simulink model "AccelerationValidation"  (R2022b)
settings: Solver=VariableStepAuto  StartTime=0.0  StopTime=10.0  RelTol=1e-3
(part 2 of 2)

== matlab function AccelerationValidation/MATLAB Function ==
  data: q input; AF output; qdot input; qdd input
function AF = forward_acceleration_kinematics(q, qdot, qdd)

q1 = q(1);
q2 = q(2);
q3 = q(3);
q4 = q(4);
q1dot = qdot(1);
q2dot = qdot(2);
q3dot = qdot(3);
q4dot = qdot(4);
q1dd = qdd(1);
q2dd = qdd(2);
q3dd = qdd(3);
q4dd = qdd(4);

J =[150*sin(q2)*sin(q1 - pi/2)*sin(q4 - pi/2) - 150*cos(q4 - pi/2)*(cos(q1 - pi/2)*sin(q3 - pi/2) + cos(q2)*cos(q3 - pi/2)*sin(q1 - pi/2)) - 185*sin(q2)*sin(q1 - pi/2),                                                                                                                                                                                                                                                                      -cos(q1 - pi/2)*(150*cos(q2)*sin(q4 - pi/2) - 185*cos(q2) + 150*cos(q3 - pi/2)*cos(q4 - pi/2)*sin(q2)),                                                                                             - cos(q2)*(185*sin(q2)*sin(q1 - pi/2) + 150*cos(q4 - pi/2)*(cos(q1 - pi/2)*sin(q3 - pi/2) + cos(q2)*cos(q3 - pi/2)*sin(q1 - pi/2)) - 150*sin(q2)*sin(q1 - pi/2)*sin(q4 - pi/2)) - sin(q2)*sin(q1 - pi/2)*(150*cos(q2)*sin(q4 - pi/2) - 185*cos(q2) + 150*cos(q3 - pi/2)*cos(q4 - pi/2)*sin(q2)),                                                                                                                - (150*cos(q2)*sin(q4 - pi/2) + 150*cos(q3 - pi/2)*cos(q4 - pi/2)*sin(q2))*(cos(q1 - pi/2)*cos(q3 - pi/2) - cos(q2)*sin(q1 - pi/2)*sin(q3 - pi/2)) - sin(q2)*sin(q3 - pi/2)*(150*cos(q4 - pi/2)*(cos(q1 - pi/2)*sin(q3 - pi/2) + cos(q2)*cos(q3 - pi/2)*sin(q1 - pi/2)) - 150*sin(q2)*sin(q1 - pi/2)*sin(q4 - pi/2));
185*cos(q1 - pi/2)*sin(q2) - 150*cos(q4 - pi/2)*(sin(q1 - pi/2)*sin(q3 - pi/2) - cos(q2)*cos(q1 - pi/2)*cos(q3 - pi/2)) - 150*cos(q1 - pi/2)*sin(q2)*sin(q4 - pi/2),                                                                                                                                                                                                                                                                      -sin(q1 - pi/2)*(150*cos(q2)*sin(q4 - pi/2) - 185*cos(q2) + 150*cos(q3 - pi/2)*cos(q4 - pi/2)*sin(q2)),                                                                                               cos(q1 - pi/2)*sin(q2)*(150*cos(q2)*sin(q4 - pi/2) - 185*cos(q2) + 150*cos(q3 - pi/2)*cos(q4 - pi/2)*sin(q2)) - cos(q2)*(150*cos(q4 - pi/2)*(sin(q1 - pi/2)*sin(q3 - pi/2) - cos(q2)*cos(q1 - pi/2)*cos(q3 - pi/2)) - 185*cos(q1 - pi/2)*sin(q2) + 150*cos(q1 - pi/2)*sin(q2)*sin(q4 - pi/2)),                                                                                                                - (150*cos(q2)*sin(q4 - pi/2) + 150*cos(q3 - pi/2)*cos(q4 - pi/2)*sin(q2))*(cos(q3 - pi/2)*sin(q1 - pi/2) + cos(q2)*cos(q1 - pi/2)*sin(q3 - pi/2)) - sin(q2)*sin(q3 - pi/2)*(150*cos(q4 - pi/2)*(sin(q1 - pi/2)*sin(q3 - pi/2) - cos(q2)*cos(q1 - pi/2)*cos(q3 - pi/2)) + 150*cos(q1 - pi/2)*sin(q2)*sin(q4 - pi/2));
                                                                                                                                                                  0, cos(q1 - pi/2)*(150*cos(q4 - pi/2)*(sin(q1 - pi/2)*sin(q3 - pi/2) - cos(q2)*cos(q1 - pi/2)*cos(q3 - pi/2)) - 185*cos(q1 - pi/2)*sin(q2) + 150*cos(q1 - pi/2)*sin(q2)*sin(q4 - pi/2)) - sin(q1 - pi/2)*(185*sin(q2)*sin(q1 - pi/2) + 150*cos(q4 - pi/2)*(cos(q1 - pi/2)*sin(q3 - pi/2) + cos(q2)*cos(q3 - pi/2)*sin(q1 - pi/2)) - 150*sin(q2)*sin(q1 - pi/2)*sin(q4 - pi/2)), sin(q2)*sin(q1 - pi/2)*(150*cos(q4 - pi/2)*(sin(q1 - pi/2)*sin(q3 - pi/2) - cos(q2)*cos(q1 - pi/2)*cos(q3 - pi/2)) - 185*cos(q1 - pi/2)*sin(q2) + 150*cos(q1 - pi/2)*sin(q2)*sin(q4 - pi/2)) + cos(q1 - pi/2)*sin(q2)*(185*sin(q2)*sin(q1 - pi/2) + 150*cos(q4 - pi/2)*(cos(q1 - pi/2)*sin(q3 - pi/2) + cos(q2)*cos(q3 - pi/2)*sin(q1 - pi/2)) - 150*sin(q2)*sin(q1 - pi/2)*sin(q4 - pi/2)), (150*cos(q4 - pi/2)*(sin(q1 - pi/2)*sin(q3 - pi/2) - cos(q2)*cos(q1 - pi/2)*cos(q3 - pi/2)) + 150*cos(q1 - pi/2)*sin(q2)*sin(q4 - pi/2))*(cos(q1 - pi/2)*cos(q3 - pi/2) - cos(q2)*sin(q1 - pi/2)*sin(q3 - pi/2)) - (150*cos(q4 - pi/2)*(cos(q1 - pi/2)*sin(q3 - pi/2) + cos(q2)*cos(q3 - pi/2)*sin(q1 - pi/2)) - 150*sin(q2)*sin(q1 - pi/2)*sin(q4 - pi/2))*(cos(q3 - pi/2)*sin(q1 - pi/2) + cos(q2)*cos(q1 - pi/2)*sin(q3 - pi/2));
                                                                                                                                                                  0,                                                                                                                                                                                                                                                                                                                                                             -sin(q1 - pi/2),                                                                                                                                                                                                                                                                                                                                                                      cos(q1 - pi/2)*sin(q2),                                                                                                                                                                                                                                                                                                                                                             - cos(q3 - pi/2)*sin(q1 - pi/2) - cos(q2)*cos(q1 - pi/2)*sin(q3 - pi/2);
                                                                                                                                                                  0,                                                                                                                                                                                                                                                                                                                                                              cos(q1 - pi/2),                                                                                                                                                                                                                                                                                                                                                                      sin(q2)*sin(q1 - pi/2),                                                                                                                                                                                                                                                                                                                                                               cos(q1 - pi/2)*cos(q3 - pi/2) - cos(q2)*sin(q1 - pi/2)*sin(q3 - pi/2);                                                                                                                                                                  1,                                                                                                                                                                                                                                                                                                                                                                           0,                                                                                                                                                                                                                                                                                                                                                                                     cos(q2),                                                                                                                                                                                                                                                                                                                                                                                                              sin(q2)*sin(q3 - pi/2)];
 
J_dot = [q4dot*(150*sin(q4 - pi/2)*(cos(q1 - pi/2)*sin(q3 - pi/2) + cos(q2)*cos(q3 - pi/2)*sin(q1 - pi/2)) + 150*cos(q4 - pi/2)*sin(q2)*sin(q1 - pi/2)) + q1dot*(150*cos(q4 - pi/2)*(sin(q1 - pi/2)*sin(q3 - pi/2) - cos(q2)*cos(q1 - pi/2)*cos(q3 - pi/2)) - 185*cos(q1 - pi/2)*sin(q2) + 150*cos(q1 - pi/2)*sin(q2)*sin(q4 - pi/2)) + q2dot*(150*cos(q2)*sin(q1 - pi/2)*sin(q4 - pi/2) - 185*cos(q2)*sin(q1 - pi/2) + 150*cos(q3 - pi/2)*cos(q4 - pi/2)*sin(q2)*sin(q1 - pi/2)) - 150*q3dot*cos(q4 - pi/2)*(cos(q1 - pi/2)*cos(q3 - pi/2) - cos(q2)*sin(q1 - pi/2)*sin(q3 - pi/2)),                                                                                                                                                                                                                                                                                                                                                                                                                                                                                  q1dot*sin(q1 - pi/2)*(150*cos(q2)*sin(q4 - pi/2) - 185*cos(q2) + 150*cos(q3 - pi/2)*cos(q4 - pi/2)*sin(q2)) - q4dot*cos(q1 - pi/2)*(150*cos(q2)*cos(q4 - pi/2) - 150*cos(q3 - pi/2)*sin(q2)*sin(q4 - pi/2)) - q2dot*cos(q1 - pi/2)*(185*sin(q2) - 150*sin(q2)*sin(q4 - pi/2) + 150*cos(q2)*cos(q3 - pi/2)*cos(q4 - pi/2)) + 150*q3dot*cos(q1 - pi/2)*cos(q4 - pi/2)*sin(q2)*sin(q3 - pi/2),        q4dot*(cos(q2)*(150*sin(q4 - pi/2)*(cos(q1 - pi/2)*sin(q3 - pi/2) + cos(q2)*cos(q3 - pi/2)*sin(q1 - pi/2)) + 150*cos(q4 - pi/2)*sin(q2)*sin(q1 - pi/2)) - sin(q2)*sin(q1 - pi/2)*(150*cos(q2)*cos(q4 - pi/2) - 150*cos(q3 - pi/2)*sin(q2)*sin(q4 - pi/2))) - q3dot*(150*cos(q2)*cos(q4 - pi/2)*(cos(q1 - pi/2)*cos(q3 - pi/2) - cos(q2)*sin(q1 - pi/2)*sin(q3 - pi/2)) - 150*cos(q4 - pi/2)*sin(q2)^2*sin(q1 - pi/2)*sin(q3 - pi/2)) + q1dot*(cos(q2)*(150*cos(q4 - pi/2)*(sin(q1 - pi/2)*sin(q3 - pi/2) - cos(q2)*cos(q1 - pi/2)*cos(q3 - pi/2)) - 185*cos(q1 - pi/2)*sin(q2) + 150*cos(q1 - pi/2)*sin(q2)*sin(q4 - pi/2)) - cos(q1 - pi/2)*sin(q2)*(150*cos(q2)*sin(q4 - pi/2) - 185*cos(q2) + 150*cos(q3 - pi/2)*cos(q4 - pi/2)*sin(q2))) + q2dot*(cos(q2)*(150*cos(q2)*sin(q1 - pi/2)*sin(q4 - pi/2) - 185*cos(q2)*sin(q1 - pi/2) + 150*cos(q3 - pi/2)*cos(q4 - pi/2)*sin(q2)*sin(q1 - pi/2)) + sin(q2)*(185*sin(q2)*sin(q1 - pi/2) + 150*cos(q4 - pi/2)*(cos(q1 - pi/2)*sin(q3 - pi/2) + cos(q2)*cos(q3 - pi/2)*sin(q1 - pi/2)) - 150*sin(q2)*sin(q1 - pi/2)*sin(q4 - pi/2)) - sin(q2)*sin(q1 - pi/2)*(185*sin(q2) - 150*sin(q2)*sin(q4 - pi/2) + 150*cos(q2)*cos(q3 - pi/2)*cos(q4 - pi/2)) - cos(q2)*sin(q1 - pi/2)*(150*cos(q2)*sin(q4 - pi/2) - 185*cos(q2) + 150*cos(q3 - pi/2)*cos(q4 - pi/2)*sin(q2))),                                                                    q1dot*((150*cos(q2)*sin(q4 - pi/2) + 150*cos(q3 - pi/2)*cos(q4 - pi/2)*sin(q2))*(cos(q3 - pi/2)*sin(q1 - pi/2) + cos(q2)*cos(q1 - pi/2)*sin(q3 - pi/2)) + sin(q2)*sin(q3 - pi/2)*(150*cos(q4 - pi/2)*(sin(q1 - pi/2)*sin(q3 - pi/2) - cos(q2)*cos(q1 - pi/2)*cos(q3 - pi/2)) + 150*cos(q1 - pi/2)*sin(q2)*sin(q4 - pi/2))) + q3dot*((150*cos(q2)*sin(q4 - pi/2) + 150*cos(q3 - pi/2)*cos(q4 - pi/2)*sin(q2))*(cos(q1 - pi/2)*sin(q3 - pi/2) + cos(q2)*cos(q3 - pi/2)*sin(q1 - pi/2)) - cos(q3 - pi/2)*sin(q2)*(150*cos(q4 - pi/2)*(cos(q1 - pi/2)*sin(q3 - pi/2) + cos(q2)*cos(q3 - pi/2)*sin(q1 - pi/2)) - 150*sin(q2)*sin(q1 - pi/2)*sin(q4 - pi/2))) - q4dot*((150*cos(q2)*cos(q4 - pi/2) - 150*cos(q3 - pi/2)*sin(q2)*sin(q4 - pi/2))*(cos(q1 - pi/2)*cos(q3 - pi/2) - cos(q2)*sin(q1 - pi/2)*sin(q3 - pi/2)) - sin(q2)*sin(q3 - pi/2)*(150*sin(q4 - pi/2)*(cos(q1 - pi/2)*sin(q3 - pi/2) + cos(q2)*cos(q3 - pi/2)*sin(q1 - pi/2)) + 150*cos(q4 - pi/2)*sin(q2)*sin(q1 - pi/2))) + q2dot*((150*sin(q2)*sin(q4 - pi/2) - 150*cos(q2)*cos(q3 - pi/2)*cos(q4 - pi/2))*(cos(q1 - pi/2)*cos(q3 - pi/2) - cos(q2)*sin(q1 - pi/2)*sin(q3 - pi/2)) - cos(q2)*sin(q3 - pi/2)*(150*cos(q4 - pi/2)*(cos(q1 - pi/2)*sin(q3 - pi/2) + cos(q2)*cos(q3 - pi/2)*sin(q1 - pi/2)) - 150*sin(q2)*sin(q1 - pi/2)*sin(q4 - pi/2)) + sin(q2)*sin(q3 - pi/2)*(150*cos(q2)*sin(q1 - pi/2)*sin(q4 - pi/2) + 150*cos(q3 - pi/2)*cos(q4 - pi/2)*sin(q2)*sin(q1 - pi/2)) - sin(q2)*sin(q1 - pi/2)*sin(q3 - pi/2)*(150*cos(q2)*sin(q4 - pi/2) + 150*cos(q3 - pi/2)*cos(q4 - pi/2)*sin(q2)));
q4dot*(150*sin(q4 - pi/2)*(sin(q1 - pi/2)*sin(q3 - pi/2) - cos(q2)*cos(q1 - pi/2)*cos(q3 - pi/2)) - 150*cos(q1 - pi/2)*cos(q4 - pi/2)*sin(q2)) - q2dot*(150*cos(q2)*cos(q1 - pi/2)*sin(q4 - pi/2) - 185*cos(q2)*cos(q1 - pi/2) + 150*cos(q1 - pi/2)*cos(q3 - pi/2)*cos(q4 - pi/2)*sin(q2)) - q1dot*(185*sin(q2)*sin(q1 - pi/2) + 150*cos(q4 - pi/2)*(cos(q1 - pi/2)*sin(q3 - pi/2) + cos(q2)*cos(q3 - pi/2)*sin(q1 - pi/2)) - 150*sin(q2)*sin(q1 - pi/2)*sin(q4 - pi/2)) - 150*q3dot*cos(q4 - pi/2)*(cos(q3 - pi/2)*sin(q1 - pi/2) + cos(q2)*cos(q1 - pi/2)*sin(q3 - pi/2)),                                                                                                                                                                                                                                                                                                                                                                                                                                                                                  150*q3dot*cos(q4 - pi/2)*sin(q2)*sin(q1 - pi/2)*sin(q3 - pi/2) - q1dot*cos(q1 - pi/2)*(150*cos(q2)*sin(q4 - pi/2) - 185*cos(q2) + 150*cos(q3 - pi/2)*cos(q4 - pi/2)*sin(q2)) - q2dot*sin(q1 - pi/2)*(185*sin(q2) - 150*sin(q2)*sin(q4 - pi/2) + 150*cos(q2)*cos(q3 - pi/2)*cos(q4 - pi/2)) - q4dot*sin(q1 - pi/2)*(150*cos(q2)*cos(q4 - pi/2) - 150*cos(q3 - pi/2)*sin(q2)*sin(q4 - pi/2)),        q2dot*(sin(q2)*(150*cos(q4 - pi/2)*(sin(q1 - pi/2)*sin(q3 - pi/2) - cos(q2)*cos(q1 - pi/2)*cos(q3 - pi/2)) - 185*cos(q1 - pi/2)*sin(q2) + 150*cos(q1 - pi/2)*sin(q2)*sin(q4 - pi/2)) - cos(q2)*(150*cos(q2)*cos(q1 - pi/2)*sin(q4 - pi/2) - 185*cos(q2)*cos(q1 - pi/2) + 150*cos(q1 - pi/2)*cos(q3 - pi/2)*cos(q4 - pi/2)*sin(q2)) + cos(q2)*cos(q1 - pi/2)*(150*cos(q2)*sin(q4 - pi/2) - 185*cos(q2) + 150*cos(q3 - pi/2)*cos(q4 - pi/2)*sin(q2)) + cos(q1 - pi/2)*sin(q2)*(185*sin(q2) - 150*sin(q2)*sin(q4 - pi/2) + 150*cos(q2)*cos(q3 - pi/2)*cos(q4 - pi/2))) - q3dot*(150*cos(q2)*cos(q4 - pi/2)*(cos(q3 - pi/2)*sin(q1 - pi/2) + cos(q2)*cos(q1 - pi/2)*sin(q3 - pi/2)) + 150*cos(q1 - pi/2)*cos(q4 - pi/2)*sin(q2)^2*sin(q3 - pi/2)) - q1dot*(cos(q2)*(185*sin(q2)*sin(q1 - pi/2) + 150*cos(q4 - pi/2)*(cos(q1 - pi/2)*sin(q3 - pi/2) + cos(q2)*cos(q3 - pi/2)*sin(q1 - pi/2)) - 150*sin(q2)*sin(q1 - pi/2)*sin(q4 - pi/2)) + sin(q2)*sin(q1 - pi/2)*(150*cos(q2)*sin(q4 - pi/2) - 185*cos(q2) + 150*cos(q3 - pi/2)*cos(q4 - pi/2)*sin(q2))) + q4dot*(cos(q2)*(150*sin(q4 - pi/2)*(sin(q1 - pi/2)*sin(q3 - pi/2) - cos(q2)*cos(q1 - pi/2)*cos(q3 - pi/2)) - 150*cos(q1 - pi/2)*cos(q4 - pi/2)*sin(q2)) + cos(q1 - pi/2)*sin(q2)*(150*cos(q2)*cos(q4 - pi/2) - 150*cos(q3 - pi/2)*sin(q2)*sin(q4 - pi/2))),                                                                    q3dot*((150*cos(q2)*sin(q4 - pi/2) + 150*cos(q3 - pi/2)*cos(q4 - pi/2)*sin(q2))*(sin(q1 - pi/2)*sin(q3 - pi/2) - cos(q2)*cos(q1 - pi/2)*cos(q3 - pi/2)) - cos(q3 - pi/2)*sin(q2)*(150*cos(q4 - pi/2)*(sin(q1 - pi/2)*sin(q3 - pi/2) - cos(q2)*cos(q1 - pi/2)*cos(q3 - pi/2)) + 150*cos(q1 - pi/2)*sin(q2)*sin(q4 - pi/2))) - q4dot*((150*cos(q2)*cos(q4 - pi/2) - 150*cos(q3 - pi/2)*sin(q2)*sin(q4 - pi/2))*(cos(q3 - pi/2)*sin(q1 - pi/2) + cos(q2)*cos(q1 - pi/2)*sin(q3 - pi/2)) - sin(q2)*sin(q3 - pi/2)*(150*sin(q4 - pi/2)*(sin(q1 - pi/2)*sin(q3 - pi/2) - cos(q2)*cos(q1 - pi/2)*cos(q3 - pi/2)) - 150*cos(q1 - pi/2)*cos(q4 - pi/2)*sin(q2))) - q1dot*((150*cos(q2)*sin(q4 - pi/2) + 150*cos(q3 - pi/2)*cos(q4 - pi/2)*sin(q2))*(cos(q1 - pi/2)*cos(q3 - pi/2) - cos(q2)*sin(q1 - pi/2)*sin(q3 - pi/2)) + sin(q2)*sin(q3 - pi/2)*(150*cos(q4 - pi/2)*(cos(q1 - pi/2)*sin(q3 - pi/2) + cos(q2)*cos(q3 - pi/2)*sin(q1 - pi/2)) - 150*sin(q2)*sin(q1 - pi/2)*sin(q4 - pi/2))) + q2dot*((150*sin(q2)*sin(q4 - pi/2) - 150*cos(q2)*cos(q3 - pi/2)*cos(q4 - pi/2))*(cos(q3 - pi/2)*sin(q1 - pi/2) + cos(q2)*cos(q1 - pi/2)*sin(q3 - pi/2)) - cos(q2)*sin(q3 - pi/2)*(150*cos(q4 - pi/2)*(sin(q1 - pi/2)*sin(q3 - pi/2) - cos(q2)*cos(q1 - pi/2)*cos(q3 - pi/2)) + 150*cos(q1 - pi/2)*sin(q2)*sin(q4 - pi/2)) - sin(q2)*sin(q3 - pi/2)*(150*cos(q2)*cos(q1 - pi/2)*sin(q4 - pi/2) + 150*cos(q1 - pi/2)*cos(q3 - pi/2)*cos(q4 - pi/2)*sin(q2)) + cos(q1 - pi/2)*sin(q2)*sin(q3 - pi/2)*(150*cos(q2)*sin(q4 - pi/2) + 150*cos(q3 - pi/2)*cos(q4 - pi/2)*sin(q2)));
                                                                                                                                                                                                                                                                                                                                                                                                                                                                                                                                                                          0, q3dot*(150*cos(q1 - pi/2)*cos(q4 - pi/2)*(cos(q3 - pi/2)*sin(q1 - pi/2) + cos(q2)*cos(q1 - pi/2)*sin(q3 - pi/2)) - 150*cos(q4 - pi/2)*sin(q1 - pi/2)*(cos(q1 - pi/2)*cos(q3 - pi/2) - cos(q2)*sin(q1 - pi/2)*sin(q3 - pi/2))) - q4dot*(cos(q1 - pi/2)*(150*sin(q4 - pi/2)*(sin(q1 - pi/2)*sin(q3 - pi/2) - cos(q2)*cos(q1 - pi/2)*cos(q3 - pi/2)) - 150*cos(q1 - pi/2)*cos(q4 - pi/2)*sin(q2)) - sin(q1 - pi/2)*(150*sin(q4 - pi/2)*(cos(q1 - pi/2)*sin(q3 - pi/2) + cos(q2)*cos(q3 - pi/2)*sin(q1 - pi/2)) + 150*cos(q4 - pi/2)*sin(q2)*sin(q1 - pi/2))) + q2dot*(cos(q1 - pi/2)*(150*cos(q2)*cos(q1 - pi/2)*sin(q4 - pi/2) - 185*cos(q2)*cos(q1 - pi/2) + 150*cos(q1 - pi/2)*cos(q3 - pi/2)*cos(q4 - pi/2)*sin(q2)) + sin(q1 - pi/2)*(150*cos(q2)*sin(q1 - pi/2)*sin(q4 - pi/2) - 185*cos(q2)*sin(q1 - pi/2) + 150*cos(q3 - pi/2)*cos(q4 - pi/2)*sin(q2)*sin(q1 - pi/2))), q2dot*(sin(q2)*sin(q1 - pi/2)*(150*cos(q2)*cos(q1 - pi/2)*sin(q4 - pi/2) - 185*cos(q2)*cos(q1 - pi/2) + 150*cos(q1 - pi/2)*cos(q3 - pi/2)*cos(q4 - pi/2)*sin(q2)) + cos(q2)*sin(q1 - pi/2)*(150*cos(q4 - pi/2)*(sin(q1 - pi/2)*sin(q3 - pi/2) - cos(q2)*cos(q1 - pi/2)*cos(q3 - pi/2)) - 185*cos(q1 - pi/2)*sin(q2) + 150*cos(q1 - pi/2)*sin(q2)*sin(q4 - pi/2)) + cos(q2)*cos(q1 - pi/2)*(185*sin(q2)*sin(q1 - pi/2) + 150*cos(q4 - pi/2)*(cos(q1 - pi/2)*sin(q3 - pi/2) + cos(q2)*cos(q3 - pi/2)*sin(q1 - pi/2)) - 150*sin(q2)*sin(q1 - pi/2)*sin(q4 - pi/2)) - cos(q1 - pi/2)*sin(q2)*(150*cos(q2)*sin(q1 - pi/2)*sin(q4 - pi/2) - 185*cos(q2)*sin(q1 - pi/2) + 150*cos(q3 - pi/2)*cos(q4 - pi/2)*sin(q2)*sin(q1 - pi/2))) - q4dot*(cos(q1 - pi/2)*sin(q2)*(150*sin(q4 - pi/2)*(cos(q1 - pi/2)*sin(q3 - pi/2) + cos(q2)*cos(q3 - pi/2)*sin(q1 - pi/2)) + 150*cos(q4 - pi/2)*sin(q2)*sin(q1 - pi/2)) + sin(q2)*sin(q1 - pi/2)*(150*sin(q4 - pi/2)*(sin(q1 - pi/2)*sin(q3 - pi/2) - cos(q2)*cos(q1 - pi/2)*cos(q3 - pi/2)) - 150*cos(q1 - pi/2)*cos(q4 - pi/2)*sin(q2))) + q3dot*(150*cos(q1 - pi/2)*cos(q4 - pi/2)*sin(q2)*(cos(q1 - pi/2)*cos(q3 - pi/2) - cos(q2)*sin(q1 - pi/2)*sin(q3 - pi/2)) + 150*cos(q4 - pi/2)*sin(q2)*sin(q1 - pi/2)*(cos(q3 - pi/2)*sin(q1 - pi/2) + cos(q2)*cos(q1 - pi/2)*sin(q3 - pi/2))), q2dot*((150*cos(q2)*cos(q1 - pi/2)*sin(q4 - pi/2) + 150*cos(q1 - pi/2)*cos(q3 - pi/2)*cos(q4 - pi/2)*sin(q2))*(cos(q1 - pi/2)*cos(q3 - pi/2) - cos(q2)*sin(q1 - pi/2)*sin(q3 - pi/2)) + (150*cos(q2)*sin(q1 - pi/2)*sin(q4 - pi/2) + 150*cos(q3 - pi/2)*cos(q4 - pi/2)*sin(q2)*sin(q1 - pi/2))*(cos(q3 - pi/2)*sin(q1 - pi/2) + cos(q2)*cos(q1 - pi/2)*sin(q3 - pi/2)) + cos(q1 - pi/2)*sin(q2)*sin(q3 - pi/2)*(150*cos(q4 - pi/2)*(cos(q1 - pi/2)*sin(q3 - pi/2) + cos(q2)*cos(q3 - pi/2)*sin(q1 - pi/2)) - 150*sin(q2)*sin(q1 - pi/2)*sin(q4 - pi/2)) + sin(q2)*sin(q1 - pi/2)*sin(q3 - pi/2)*(150*cos(q4 - pi/2)*(sin(q1 - pi/2)*sin(q3 - pi/2) - cos(q2)*cos(q1 - pi/2)*cos(q3 - pi/2)) + 150*cos(q1 - pi/2)*sin(q2)*sin(q4 - pi/2))) - q3dot*((150*cos(q4 - pi/2)*(sin(q1 - pi/2)*sin(q3 - pi/2) - cos(q2)*cos(q1 - pi/2)*cos(q3 - pi/2)) + 150*cos(q1 - pi/2)*sin(q2)*sin(q4 - pi/2))*(cos(q1 - pi/2)*sin(q3 - pi/2) + cos(q2)*cos(q3 - pi/2)*sin(q1 - pi/2)) - (150*cos(q4 - pi/2)*(cos(q1 - pi/2)*sin(q3 - pi/2) + cos(q2)*cos(q3 - pi/2)*sin(q1 - pi/2)) - 150*sin(q2)*sin(q1 - pi/2)*sin(q4 - pi/2))*(sin(q1 - pi/2)*sin(q3 - pi/2) - cos(q2)*cos(q1 - pi/2)*cos(q3 - pi/2))) - q4dot*((150*sin(q4 - pi/2)*(sin(q1 - pi/2)*sin(q3 - pi/2) - cos(q2)*cos(q1 - pi/2)*cos(q3 - pi/2)) - 150*cos(q1 - pi/2)*cos(q4 - pi/2)*sin(q2))*(cos(q1 - pi/2)*cos(q3 - pi/2) - cos(q2)*sin(q1 - pi/2)*sin(q3 - pi/2)) - (150*sin(q4 - pi/2)*(cos(q1 - pi/2)*sin(q3 - pi/2) + cos(q2)*cos(q3 - pi/2)*sin(q1 - pi/2)) + 150*cos(q4 - pi/2)*sin(q2)*sin(q1 - pi/2))*(cos(q3 - pi/2)*sin(q1 - pi/2) + cos(q2)*cos(q1 - pi/2)*sin(q3 - pi/2)));
                                                                                                                                                                                                                                                                                                                                                                                                                                                                                                                                                                          0,                                                                                                                                                                                                                                                                                                                                                                                                                                                                                                                                                                                                                                                                                                                                                                                                                                                       -q1dot*cos(q1 - pi/2),                                                                                                                                                                                                                                                                                                                                                                                                                                                                                                                                                                                                                                                                                                                                                                                                                                                                                                                                                                                                                                                                                                                                                                                                                                                               q2dot*cos(q2)*cos(q1 - pi/2) - q1dot*sin(q2)*sin(q1 - pi/2),                                                                                                                                                                                                                                                                                                                                                                                                                                                                                                                                                                                                                                                                                                                                                                                                                                                                                                                                                                                                                                                                                                                                                                                                                                                                                                                                                                                                                           q3dot*(sin(q1 - pi/2)*sin(q3 - pi/2) - cos(q2)*cos(q1 - pi/2)*cos(q3 - pi/2)) - q1dot*(cos(q1 - pi/2)*cos(q3 - pi/2) - cos(q2)*sin(q1 - pi/2)*sin(q3 - pi/2)) + q2dot*cos(q1 - pi/2)*sin(q2)*sin(q3 - pi/2);
                                                                                                                                                                                                                                                                                                                                                                                                                                                                                                                                                                          0,                                                                                                                                                                                                                                                                                                                                                                                                                                                                                                                                                                                                                                                                                                                                                                                                                                                       -q1dot*sin(q1 - pi/2),                                                                                                                                                                                                                                                                                                                                                                                                                                                                                                                                                                                                                                                                                                                                                                                                                                                                                                                                                                                                                                                                                                                                                                                                                                                               q1dot*cos(q1 - pi/2)*sin(q2) + q2dot*cos(q2)*sin(q1 - pi/2),                                                                                                                                                                                                                                                                                                                                                                                                                                                                                                                                                                                                                                                                                                                                                                                                                                                                                                                                                                                                                                                                                                                                                                                                                                                                                                                                                                                                                           q2dot*sin(q2)*sin(q1 - pi/2)*sin(q3 - pi/2) - q3dot*(cos(q1 - pi/2)*sin(q3 - pi/2) + cos(q2)*cos(q3 - pi/2)*sin(q1 - pi/2)) - q1dot*(cos(q3 - pi/2)*sin(q1 - pi/2) + cos(q2)*cos(q1 - pi/2)*sin(q3 - pi/2));
                                                                                                                                                                                                                                                                                                                                                                                                                                                                                                                                                                          0,                                                                                                                                                                                                                                                                                                                                                                                                                                                                                                                                                                                                                                                                                                                                                                                                                                                                           0,                                                                                                                                                                                                                                                                                                                                                                                                                                                                                                                                                                                                                                                                                                                                                                                                                                                                                                                                                                                                                                                                                                                                                                                                                                                                                                            -q2dot*sin(q2),                                                                                                                                                                                                                                                                                                                                                                                                                                                                                                                                                                                                                                                                                                                                                                                                                                                                                                                                                                                                                                                                                                                                                                                                                                                                                                                                                                                                                                                                                                                                                                           q2dot*cos(q2)*sin(q3 - pi/2) + q3dot*cos(q3 - pi/2)*sin(q2)];
 
AF = J_dot * [q1dot; q2dot; q3dot; q4dot] + J * [q1dd; q2dd; q3dd; q4dd];

end
